simulink model "two_states_with_trigger"  (R2017b)
settings: Solver=FixedStepDiscrete  StartTime=0.0  StopTime=10.0  RelTol=1e-3
settings Model: Creator=flosch  LastModifiedBy=flosch
settings ConfigComp: CovScope=ReferencedModels  CovIncludeTopModel=off

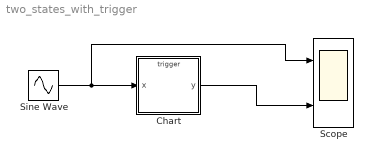
== system two_states_with_trigger ==
  Chart : Stateflow chart  TreatAsAtomicUnit=on
  Scope : Scope  NumInputPorts=2
  Sine Wave : Sin  SampleTime=0
  wires:
  Sine Wave/1 -> Scope/1, Chart/1(x)
  Chart/1(y) -> Scope/2

== stateflow chart two_states_with_trigger/Chart ==
  state Potato
    entry: y = x;
  state Kitten
    entry: y = 0;
  note: cyc = 3
      | obj = 4
      | lines = 3
  (default) -> Potato
  Potato -> Kitten : Event_A
  data: t0 constant double =0.0; x input; y output
  events: Event_A input FUNCTION_CALL_EVENT
